simulink model "TP_6"  (R2023b)
settings: Solver=VariableStepAuto  StartTime=0.0  StopTime=0.2  RelTol=1e-3
libraries: spsIGBTDiodeLib x8, spsCurrentMeasurementLib x4, spsDCVoltageSourceLib x2, spsVoltageMeasurementLib x2, spsACCurrentSourceLib x1, spsSeriesRLCBranchLib x1, sps_lib x1
settings Model: Creator=sohayl  LastModifiedBy=sohayl
settings DataIOCC: ReturnWorkspaceOutputs=off

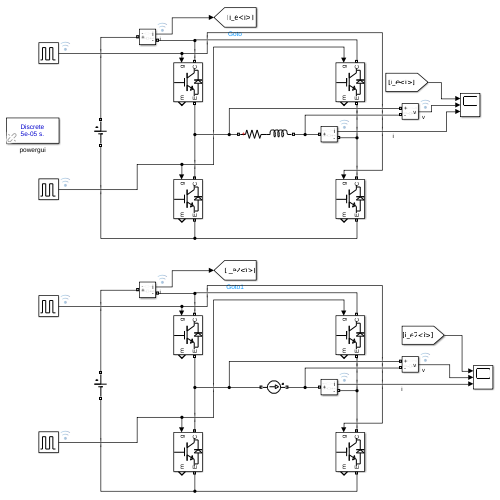
[thumbnail: Simulink's stored preview of the top-level diagram]
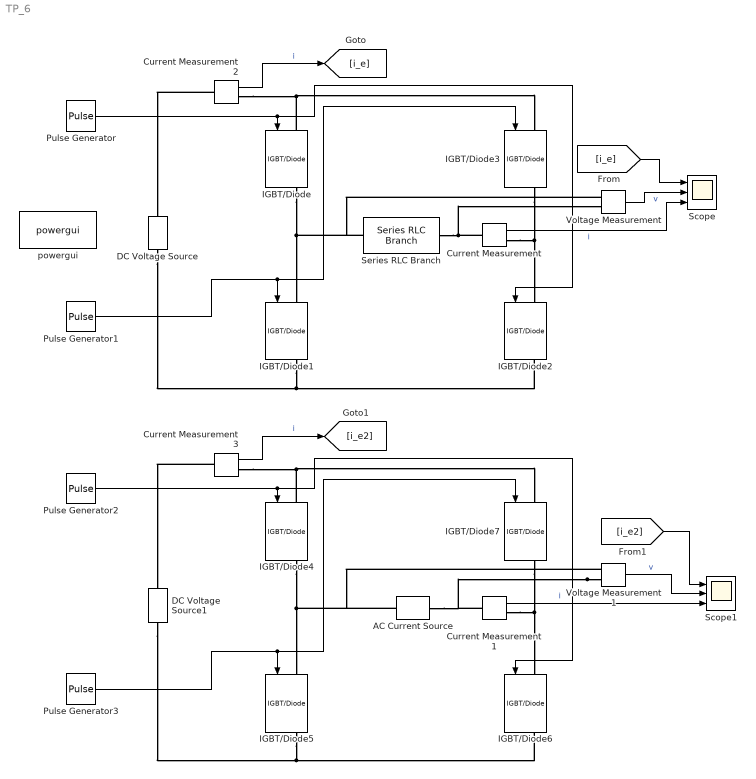
== system TP_6 ==
  AC Current Source : spsACCurrentSourceLib/AC Current Source  Amplitude=10  Phase=0  Frequency=50  SampleTime=0  Measurements=None
      settings: LibrarySourceBlock=sps_lib/Sources/AC Current Source
  Current Measurement{,1..3} (4 alike) : spsCurrentMeasurementLib/Current Measurement  PhasorSimulation=off  OutputType=Complex  PSBequivalent=0
  DC Voltage Source : spsDCVoltageSourceLib/DC Voltage Source  Amplitude=90  Measurements=None
  DC Voltage Source1 : spsDCVoltageSourceLib/DC Voltage Source  Amplitude=90  Measurements=None
  IGBT/Diode{,1..7} (8 alike) : spsIGBTDiodeLib/IGBT//Diode  Ron=1e-3  Rs=1e5  Cs=inf  Measurements=on
  Pulse Generator : DiscretePulseGenerator  PulseType=Time based  Period=0.02  PulseWidth=50
  Pulse Generator1 : DiscretePulseGenerator  PulseType=Time based  Period=0.02  PulseWidth=50  PhaseDelay=0.01
  Pulse Generator2 : DiscretePulseGenerator  PulseType=Time based  Period=0.02  PulseWidth=50
  Pulse Generator3 : DiscretePulseGenerator  PulseType=Time based  Period=0.02  PulseWidth=50  PhaseDelay=0.01
  Scope : Scope  NumInputPorts=3
  Scope1 : Scope  NumInputPorts=3
  Series RLC Branch : spsSeriesRLCBranchLib/Series RLC Branch  LConnTagsString=__new0  RConnTagsString=__new0  BranchType=RL  Resistance=10  Inductance=40e-3  SetiL0=off  InitialCurrent=0  Capacitance=1e-6  Setx0=off  InitialVoltage=0  Measurements=Branch voltage and current
  Voltage Measurement : spsVoltageMeasurementLib/Voltage Measurement  PhasorSimulation=off  OutputType=Complex  PSBequivalent=0
  Voltage Measurement1 : spsVoltageMeasurementLib/Voltage Measurement  PhasorSimulation=off  OutputType=Complex  PSBequivalent=0
  powergui : sps_lib/powergui  Priority=1  SimulationMode=Discrete  SampleTime=50e-6  frequency=60  Iterations=50  frequencyindice=0  Pbase=100e6  ErrMax=1e-4  UnitsV=kV  UnitsW=MW  buscounter=0  FunctionMessages=off  echomessages=off  EnableUseOfTLC=off  CurrentSourceSwitches=off  DisableSnubberDevices=off  DisableRonSwitches=off  DisableVfSwitches=off  DisplayEquations=off  AutomaticDiscreteSolvers=off  SolverType=Tustin/Backward Euler (TBE)  Interpol=off  ExternalGateDelay=off  methode=off  Ts=100  x0status=blocks  SPID=on  SwTol=0  HookPort=off  NonlinearTolerance=1e-4  nMaxIteration=100  ContinueOnMaxIteration=off  RestoreLinks=warning  ResistiveCurrentMeasurement=off  Frange=[0:2:500]  Ylog=off  Xlog=on  ShowGrid=off  save=off  variable=ZData  structure=0  ZoomFFT=off  StartTime=0.0  cycles=1  DisplayStyle=1  fundamental=60  FreqAxis=off  MaxFrequency=1000  frequencyindicesteady=1  RmsSteady=1  display=off
  wires:
  Pulse Generator/1 -> IGBT/Diode2/1, IGBT/Diode/1
  Pulse Generator1/1 -> IGBT/Diode3/1, IGBT/Diode1/1
  Current Measurement/1 -> Scope/3  "i"
  Pulse Generator3/1 -> IGBT/Diode7/1, IGBT/Diode5/1
  Pulse Generator2/1 -> IGBT/Diode6/1, IGBT/Diode4/1
  Current Measurement1/1 -> Scope1/3  "i"
  Voltage Measurement1/1 -> Scope1/2  "v"
  Voltage Measurement/1 -> Scope/2  "v"
  Current Measurement2/1 -> [i_e]  "i"
  [i_e] -> Scope/1
  Current Measurement3/1 -> [i_e2]  "i"
  [i_e2] -> Scope1/1
  connections:
  IGBT/Diode/RConn1 -- Voltage Measurement/LConn1 -- Series RLC Branch/LConn1 -- IGBT/Diode1/LConn1
  IGBT/Diode3/RConn1 -- Current Measurement/RConn1 -- IGBT/Diode2/LConn1
  IGBT/Diode/LConn1 -- IGBT/Diode3/LConn1 -- Current Measurement2/RConn1
  DC Voltage Source/LConn1 -- IGBT/Diode1/RConn1 -- IGBT/Diode2/RConn1
  Series RLC Branch/RConn1 -- Current Measurement/LConn1 -- Voltage Measurement/LConn2
  DC Voltage Source1/LConn1 -- IGBT/Diode5/RConn1 -- IGBT/Diode6/RConn1
  IGBT/Diode4/LConn1 -- IGBT/Diode7/LConn1 -- Current Measurement3/RConn1
  Voltage Measurement1/LConn2 -- AC Current Source/RConn1 -- Current Measurement1/LConn1
  IGBT/Diode4/RConn1 -- AC Current Source/LConn1 -- Voltage Measurement1/LConn1 -- IGBT/Diode5/LConn1
  IGBT/Diode7/RConn1 -- Current Measurement1/RConn1 -- IGBT/Diode6/LConn1
  Current Measurement2/LConn1 -- DC Voltage Source/RConn1
  Current Measurement3/LConn1 -- DC Voltage Source1/RConn1
